simulink model "CDM_simulink"  (R2020b)
settings: Solver=VariableStepAuto  StartTime=0.0  StopTime=5  RelTol=1e-3
libraries: simulink_extras x3, dspsigops x3, dsparch4 x3, commchan3 x1, commseqgen3 x1
settings Model: Creator=ASUS  LastModifiedBy=Boss Tommy
settings DataIOCC: ReturnWorkspaceOutputs=off
settings DebuggingCC: ArithmeticOperatorsInVariantConditions=warning
settings SFSimCC: SimUseLocalCustomCode=off  CustomCodeUndefinedFunction=UseInterfaceOnly
settings RTWCC: RTWUseLocalCustomCode=off

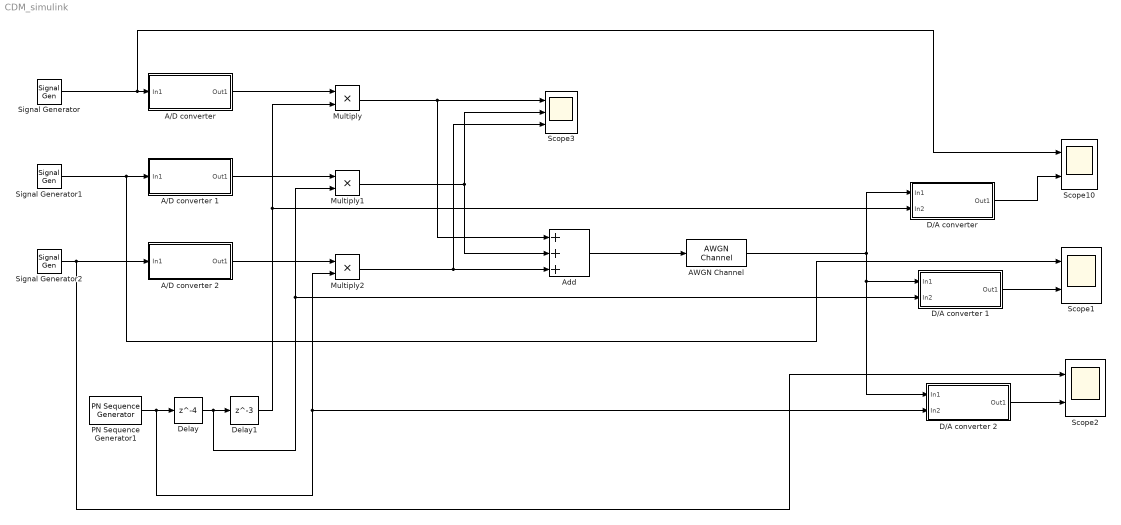
== system CDM_simulink ==
  "A/D converter " : Subsystem
  A/D converter 1 : Subsystem
  A/D converter 2 : Subsystem
  AWGN Channel : commchan3/AWGN Channel  InputProcessing=Columns as channels (frame based)  seed=67  noiseMode="Signal to noise ratio  (SNR)"  EbNodB=10  EsNodB=10  SNRdB=5  bitsPerSym=1  Ps=1  Tsym=1  variance=1
  Add : Sum  Inputs=+++
  "D/A converter " : Subsystem
  D/A converter 1 : Subsystem
  D/A converter 2 : Subsystem
  Delay : Delay  DelayLength=4  InputProcessing=Columns as channels (frame based)
  Delay1 : Delay  DelayLength=3
  Multiply : Product
  Multiply1 : Product
  Multiply2 : Product
  PN Sequence Generator1 : commseqgen3/PN Sequence Generator  poly='z^6 +z^4+z^2+z+ 1'  ini_sta=[0 0 0 0 0 1]  outBitMaskSource=Dialog parameter  shift=0  outVarSiz=off  maxOutSizeMode=Dialog parameter  maxOutSize=[10 1]  Ts=0.01  sampPerFrame=1  reset=off  bitPackedOutputs=off  outDataType=double  numPackedBits=8  bitPackDataSigned=off  bitPackedOutDType=double
  Scope1 : Scope  NumInputPorts=2
  Scope10 : Scope  NumInputPorts=2
  Scope2 : Scope  NumInputPorts=2
  Scope3 : Scope  NumInputPorts=3
  Signal Generator : SignalGenerator  Frequency=10  Units=rad/sec
  Signal Generator1 : SignalGenerator  Amplitude=2  Frequency=10  Units=rad/sec
  Signal Generator2 : SignalGenerator  Amplitude=3  Frequency=10  Units=rad/sec
  wires:
  Delay/1 -> Delay1/1, Multiply1/2, D/A converter 1/2(In2)
  A/D converter 2/1(Out1) -> Multiply2/1
  A/D converter 1/1(Out1) -> Multiply1/1
  Delay1/1 -> Multiply/2, "D/A converter "/2(In2)
  Multiply2/1 -> Scope3/3, Add/3
  Multiply1/1 -> Scope3/2, Add/2
  Multiply/1 -> Scope3/1, Add/1
  "A/D converter "/1(Out1) -> Multiply/1
  Signal Generator/1 -> Scope10/1, "A/D converter "/1(In1)
  Signal Generator1/1 -> A/D converter 1/1(In1), Scope1/1
  Signal Generator2/1 -> A/D converter 2/1(In1), Scope2/1
  Add/1 -> AWGN Channel/1
  AWGN Channel/1 -> "D/A converter "/1(In1), D/A converter 1/1(In1), D/A converter 2/1(In1)
  "D/A converter "/1(Out1) -> Scope10/2
  PN Sequence Generator1/1 -> D/A converter 2/2(In2), Multiply2/2, Delay/1
  D/A converter 1/1(Out1) -> Scope1/2
  D/A converter 2/1(Out1) -> Scope2/2

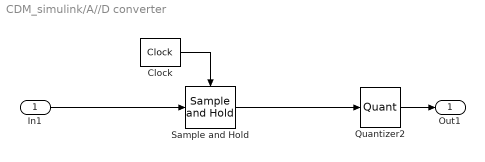
== system CDM_simulink/A//D converter  ==
  In1 : Inport
  Clock : simulink_extras/Flip Flops/Clock  period=0.01
  Quantizer2 : Quantizer  QuantizationInterval=0.2  LinearizeAsGain=off
  Sample and Hold : dspsigops/Sample and Hold  trig=Rising edge  initCond=0  latchinput=off
  Out1 : Outport  VectorParamsAs1DForOutWhenUnconnected=off
  wires:
  Clock/1 -> Sample and Hold/Trigger
  Sample and Hold/1 -> Quantizer2/1
  In1/1 -> Sample and Hold/1
  Quantizer2/1 -> Out1/1

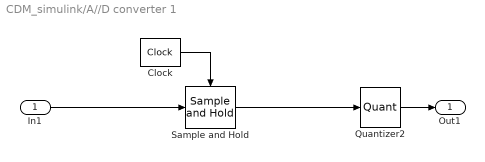
== system CDM_simulink/A//D converter 1 ==
  In1 : Inport
  Clock : simulink_extras/Flip Flops/Clock  period=0.01
  Quantizer2 : Quantizer  QuantizationInterval=0.2  LinearizeAsGain=off
  Sample and Hold : dspsigops/Sample and Hold  trig=Rising edge  initCond=0  latchinput=off
  Out1 : Outport  VectorParamsAs1DForOutWhenUnconnected=off
  wires:
  Clock/1 -> Sample and Hold/Trigger
  Sample and Hold/1 -> Quantizer2/1
  In1/1 -> Sample and Hold/1
  Quantizer2/1 -> Out1/1

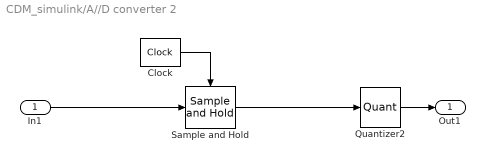
== system CDM_simulink/A//D converter 2 ==
  In1 : Inport
  Clock : simulink_extras/Flip Flops/Clock  period=0.01
  Quantizer2 : Quantizer  QuantizationInterval=0.2  LinearizeAsGain=off
  Sample and Hold : dspsigops/Sample and Hold  trig=Rising edge  initCond=0  latchinput=off
  Out1 : Outport  VectorParamsAs1DForOutWhenUnconnected=off
  wires:
  Clock/1 -> Sample and Hold/Trigger
  Sample and Hold/1 -> Quantizer2/1
  In1/1 -> Sample and Hold/1
  Quantizer2/1 -> Out1/1

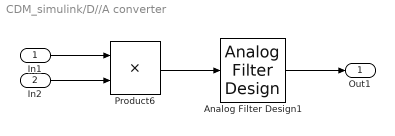
== system CDM_simulink/D//A converter  ==
  In1 : Inport
  In2 : Inport  Port=2
  Analog Filter Design1 : dsparch4/Analog Filter Design  method=Bessel  filttype=Lowpass  N=4  Wlo=20  Whi=80  Rp=2  Rs=40
  Product6 : Product
  Out1 : Outport  VectorParamsAs1DForOutWhenUnconnected=off
  wires:
  Product6/1 -> Analog Filter Design1/1
  Analog Filter Design1/1 -> Out1/1
  In1/1 -> Product6/1
  In2/1 -> Product6/2

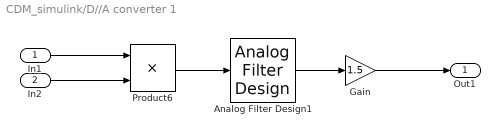
== system CDM_simulink/D//A converter 1 ==
  In1 : Inport
  In2 : Inport  Port=2
  Analog Filter Design1 : dsparch4/Analog Filter Design  method=Bessel  filttype=Lowpass  N=4  Wlo=20  Whi=80  Rp=2  Rs=40
  Gain : Gain  Gain=1.5
  Product6 : Product
  Out1 : Outport  VectorParamsAs1DForOutWhenUnconnected=off
  wires:
  Product6/1 -> Analog Filter Design1/1
  Analog Filter Design1/1 -> Gain/1
  In1/1 -> Product6/1
  In2/1 -> Product6/2
  Gain/1 -> Out1/1

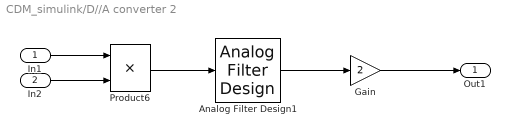
== system CDM_simulink/D//A converter 2 ==
  In1 : Inport
  In2 : Inport  Port=2
  Analog Filter Design1 : dsparch4/Analog Filter Design  method=Bessel  filttype=Lowpass  N=4  Wlo=20  Whi=80  Rp=2  Rs=40
  Gain : Gain  Gain=2
  Product6 : Product
  Out1 : Outport  VectorParamsAs1DForOutWhenUnconnected=off
  wires:
  Product6/1 -> Analog Filter Design1/1
  Analog Filter Design1/1 -> Gain/1
  In1/1 -> Product6/1
  In2/1 -> Product6/2
  Gain/1 -> Out1/1
